simulink model "PE_with_Battery"  (R2024a)
settings: Solver=VariableStepAuto  StartTime=0.0  StopTime=1  RelTol=1e-3
InitFcn:
  | %% --- Rectifier Parameters ---
  | rect_V = 10             % Peak input voltage (V)
  | rect_C = 360100e-6      % Filter capacitor (F)
  | rect_R = 2.11           % Load resistance (Ohm)
  | 
  | %% --- Buck-Boost DC-DC Converter Parameters ---
  | bb_Pe = 1/25000         % PWM period (s)
  | bb_w  = 32.2           % Duty cycle (%)
  | bb_V  = 8               % Input DC voltage (V)
  | bb_L  = 22e-6           % Inductance (H)
  | bb_C  = 10000e-6        % Output capacitor (F)
  | bb_R  = 0.1203          % Load resistance (Ohm)
  | bb_Ts = 1e-6            % Solver fixed step size (s)
undefined symbols (not defined in the file): Ion, Lithium
libraries: spsSeriesRLCBranchLib x5, spsDiodeLib x5, spsMeanLib x4, spsCurrentMeasurementLib x2, spsVoltageMeasurementLib x2, spsBatteryLib x1, spsIGBTDiodeLib x1, spsACVoltageSourceLib x1, spspowerguiLib x1
settings Model: Creator=mxf1547  LastModifiedBy=mxf1547

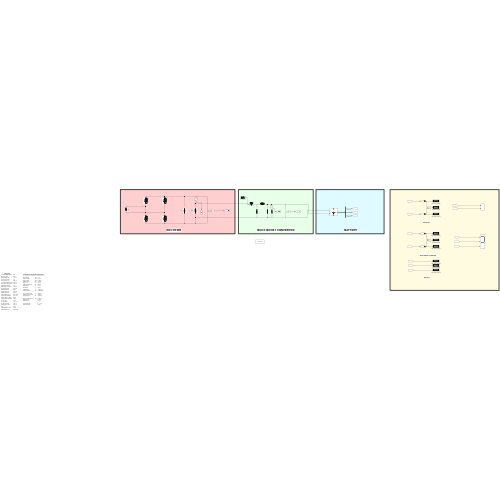
[thumbnail: Simulink's stored preview of the top-level diagram]
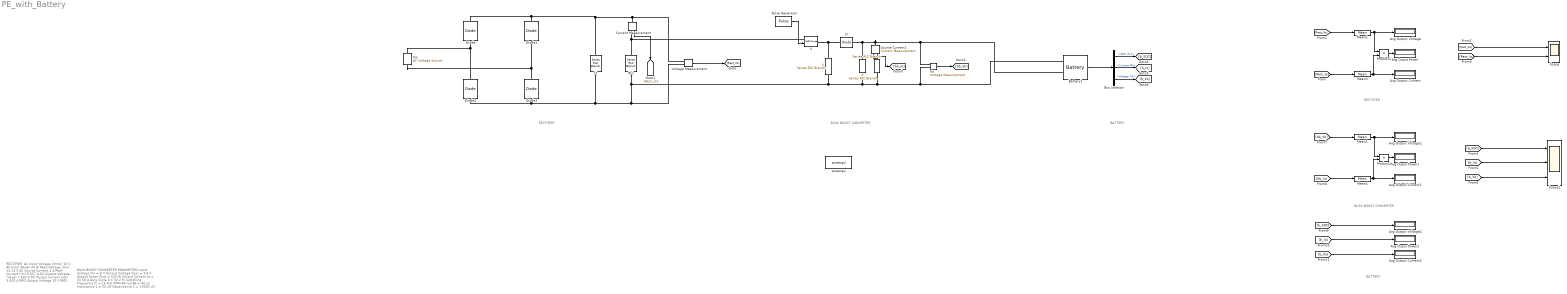
== system PE_with_Battery ==
  note: RECTIFIER
  note: BUCK-BOOST CONVERTER PARAMETERS
      |
      | Input Voltage Vin = 8 V
      | Output Voltage Vout = 3.8 V
      | Output Power Pout = 120 W
      | Output Current Ia = 31.58 A
      | Duty Cycle k = 32.2 %
      | Switching Frequency fs = 25 kHz
      | PWM Period Pe = 40 us
      |
      | Inductance L = 22 uH
      | Capacitance C = 10000 uF
      | Load Resistance R = 0.1203 Ohm
      |
      | Avg Inductor Current IL = 46.58 A
      | Peak Inductor Current = 48.92 A
      | Inductor Ripple dIL = 4.683 A
      |
      | Output Voltage Ripple dVc = 40.68 mV
      | Ripple Factor = 1.07 %
      | Voltage Stress = 11.8 V
      |
      | Solver Step Size Ts = 1 us
      | Operating Mode = CCM
  note: RECTIFIER
  note: BUCK BOOST CONVERTER
  note: RECTIFIER
      | ​
      |
      | AC Input Voltage (Vrms​)
      | 10 V
      |
      | AC Input Power
      | 40 W
      |
      | Peak Voltage (Vm​)
      | 14.14 V
      |
      | AC Source Current
      | 4 A
      |
      | Peak Current (Im​)
      | 5.657 A
      |
      | DC Output Voltage (Vavg​)
      | 7.603 V
      |
      | DC Output Current (Idc​)
      | 3.603 A
      |
      | RMS Output Voltage
      | 10 V
      |
      | RMS Output Current
      | 4.739 A
      |
      | DC Output Power
      | 27.40 W
      |
      | Rectifier Efficiency
      | 68.5%
      |
      | Diode Power Loss
      | 5.044 W
      |
      | Ripple Frequency
      | 100 Hz
      |
      | Filter Capacitor (C)
      | 360,100 μF
      |
      | Output Voltage Ripple
      | 100.1 mV
      |
      | Ripple Factor (no filter)
      | 85.5%
      |
      | Ripple Factor (with filter)
      | 0.38%
      |
      | Form Factor
      | 1.315
      |
      | PIV per Diode
      | 14.14 V
      |
      | Avg Diode Current
      | 1.801 A
      |
      | Peak Diode Current
      | 5.657 A
      |
      | TUF
      | 0.578
      |
      | Load Resistance (RL​)
      | 2.11 Ω
      |
      | Filter Capacitor (C)
      | 360,100 μF
  note: BATTERY
  note: BUCK BOOST CONVERTER
  note: BATTERY
  " " : spsSeriesRLCBranchLib/Series RLC Branch  LConnTagsString=__new0  RConnTagsString=__new0  BranchType=R  Resistance=bb_R  Inductance=1e-3  SetiL0=off  InitialCurrent=0  Capacitance=1e-6  Setx0=off  InitialVoltage=0  Measurements=None
  Avg Ouput Power : Display
  Avg Ouput Power1 : Display
  Avg Ouput Power2 : Display
  Avg Output Current : Display
  Avg Output Current1 : Display
  Avg Output Current2 : Display
  Avg Output Voltage : Display
  Avg Output Voltage1 : Display
  Avg Output Voltage2 : Display
  Battery1 : spsBatteryLib/Battery  BatType=Lithium-Ion  ShowTempParam=off  ThermalPreset=no  ShowAgeParam=off  NomV=3.8  NomQ=10  SOC=10  Batt_Tr=20  PresetModel=on  MaxQ=10  MinV=2.85  FullV=4.4232  Dis_rate=4.3478  R=0.0038  Normal_OP=9.0435  expZone="[4.1055      0.4913]"  current=[6.5 13 32.5]  Units=Time  Tci=20  NomT=20  T2=-30  MaxQ2=4.8  FullV2=7.1  Normal_OP2=5.655  expZone2="[6.58           1]"  Rca=0.6  ti=2000  Dp=0  Neq0=0  Tsim=1e6  Ta1=25  Qeol=5.4*0.9  Reol=0.013333*1.2  Char_age=[2.3478, 3]  Dis_age=[2.3478, 10]  N1=1500  N2=10500  N3=1000  N4=1400  Ta2=45  N5=950
  Bus Selector : BusSelector  OutputSignals=SOC (%),Current (A),Voltage (V)
  C : spsSeriesRLCBranchLib/Series RLC Branch  LConnTagsString=__new0  RConnTagsString=__new0  BranchType=C  Resistance=1  Inductance=1e-3  SetiL0=off  InitialCurrent=0  Capacitance=bb_C  Setx0=off  InitialVoltage=0  Measurements=None
  C1 : spsSeriesRLCBranchLib/Series RLC Branch  LConnTagsString=__new0  RConnTagsString=__new0  BranchType=C  Resistance=2.11  Inductance=50e-3  SetiL0=off  InitialCurrent=0  Capacitance=rect_C  Setx0=off  InitialVoltage=0  Measurements=Branch voltage and current
  Current Measurement : spsCurrentMeasurementLib/Current Measurement  PhasorSimulation=off  OutputType=Complex  PSBequivalent=0
  D : spsDiodeLib/Diode  Ron=0.001  Lon=0  Vf=0.001  IC=0  UseSnubber=off  Rs=500  Cs=250e-9  Measurements=off
  Diode{,1..3} (4 alike) : spsDiodeLib/Diode  Ron=0.001  Lon=0  Vf=0.8  IC=0  UseSnubber=0  Rs=500  Cs=250e-9  Measurements=off
  L : spsSeriesRLCBranchLib/Series RLC Branch  LConnTagsString=__new0  RConnTagsString=__new0  BranchType=L  Resistance=1  Inductance=bb_L  SetiL0=off  InitialCurrent=0  Capacitance=1e-6  Setx0=off  InitialVoltage=0  Measurements=None
  Mean{1..4} (4 alike) : spsMeanLib/Mean  Freq=50  Vinit=0  Ts=0
  Product1 : Product
  Product2 : Product
  Pulse Generator : DiscretePulseGenerator  PulseType=Time based  Period=bb_Pe  PulseWidth=bb_w
  RL1 : spsSeriesRLCBranchLib/Series RLC Branch  LConnTagsString=__new0  RConnTagsString=__new0  BranchType=R  Resistance=rect_R  Inductance=50e-3  SetiL0=off  InitialCurrent=0  Capacitance=1e-6  Setx0=off  InitialVoltage=0  Measurements=Branch voltage and current
  S : spsIGBTDiodeLib/IGBT//Diode  Ron=1e-3  Rs=1e5  Cs=inf  Measurements=off
  Scope : Scope  NumInputPorts=2
  Scope1 : Scope  NumInputPorts=3
  Source Current1 : spsCurrentMeasurementLib/Current Measurement  PhasorSimulation=off  OutputType=Complex  PSBequivalent=0
  Vin : spsACVoltageSourceLib/AC Voltage Source  Amplitude=rect_V  Phase=0  Frequency=50  SampleTime=0  Measurements=Voltage  BusType=swing  Pref=10e3  Qref=0  Qmin=-inf  Qmax=+inf
  Vo : spsVoltageMeasurementLib/Voltage Measurement  PhasorSimulation=off  OutputType=Complex  PSBequivalent=0
  Voltage Measurement : spsVoltageMeasurementLib/Voltage Measurement  PhasorSimulation=off  OutputType=Complex  PSBequivalent=0
  powergui : spspowerguiLib/powergui  Priority=1  SimulationMode=Continuous  SampleTime=50e-6  frequency=60  Iterations=50  frequencyindice=0  Pbase=100e6  ErrMax=1e-4  UnitsV=kV  UnitsW=MW  buscounter=0  FunctionMessages=off  echomessages=off  EnableUseOfTLC=off  CurrentSourceSwitches=off  DisableSnubberDevices=off  DisableRonSwitches=off  DisableVfSwitches=off  DisplayEquations=off  AutomaticDiscreteSolvers=off  SolverType=Tustin/Backward Euler (TBE)  Interpol=off  ExternalGateDelay=off  methode=off  Ts=100  x0status=blocks  SPID=on  SwTol=0  HookPort=off  NonlinearTolerance=1e-4  nMaxIteration=100  ContinueOnMaxIteration=off  RestoreLinks=warning  ResistiveCurrentMeasurement=off  Frange=[0:2:500]  Ylog=off  Xlog=on  ShowGrid=off  save=off  variable=ZData  structure=0  ZoomFFT=off  StartTime=0.0  cycles=1  DisplayStyle=1  fundamental=60  FreqAxis=off  MaxFrequency=1000  frequencyindicesteady=1  RmsSteady=1  display=off
  wires:
  Source Current1/1 -> [bb_Io]
  Voltage Measurement/1 -> [Rect_Vo]
  Pulse Generator/1 -> S/1
  Vo/1 -> [bb_Vo]
  Mean3/1 -> Avg Output Current/1, Product1/2
  Product1/1 -> Avg Ouput Power/1
  Mean2/1 -> Avg Output Voltage/1, Product1/1
  Current Measurement/1 -> [Rect_Io]
  Battery1/1 -> Bus Selector/1
  [Rect_Vo] -> Mean2/1
  [Rect_Io] -> Mean3/1
  [Rect_Vo] -> Scope/1
  [Rect_Io] -> Scope/2
  [bb_Io] -> Mean4/1
  [bb_Vo] -> Mean1/1
  Mean1/1 -> Product2/1, Avg Output Voltage1/1
  Product2/1 -> Avg Ouput Power1/1
  Mean4/1 -> Product2/2, Avg Output Current1/1
  Bus Selector/1 -> [b_SOC]  "<SOC (%)>"
  Bus Selector/2 -> [b_Io]  "<Current (A)>"
  Bus Selector/3 -> [b_Vo]  "<Voltage (V)>"
  [b_SOC] -> Scope1/1
  [b_Io] -> Scope1/2
  [b_Vo] -> Scope1/3
  [b_SOC] -> Avg Output Voltage2/1
  [b_Io] -> Avg Ouput Power2/1
  [b_Vo] -> Avg Output Current2/1
  connections:
  Diode1/LConn1 -- Vin/LConn1 -- Diode3/RConn1
  D/RConn1 -- L/LConn1 -- S/RConn1
  Voltage Measurement/LConn1 -- Current Measurement/LConn1 -- Diode1/RConn1 -- Diode/RConn1 -- C1/LConn1
  Battery1/LConn2 -- Source Current1/LConn1 -- C/LConn1 -- D/LConn1 -- Vo/LConn1
  " "/RConn1 -- L/RConn1 -- Voltage Measurement/LConn2 -- Diode2/LConn1 -- Diode3/LConn1 -- C1/RConn1 -- RL1/RConn1 -- C/RConn1 -- Vo/LConn2 -- Battery1/LConn1
  Diode/LConn1 -- Vin/RConn1 -- Diode2/RConn1
  Current Measurement/RConn1 -- RL1/LConn1 -- S/LConn1
  Source Current1/RConn1 -- " "/LConn1
